simulink model "hvac_1zone_v3"  (R2021a)
settings: Solver=ode45  StartTime=0.0  StopTime=3600*24*3  FixedStep=2  RelTol=1e-3  EnableMultiTasking=on
undefined symbols (not defined in the file or in its folder): den, num, params1, rl
libraries: rllib x1
settings Model: Creator=User  LastModifiedBy=Richi
settings SolverCC: AlgebraicLoopSolver=TrustRegion
settings DataIOCC: LimitDataPoints=on  SaveFormat=Array  SignalLoggingSaveFormat=ModelDataLogs  ReturnWorkspaceOutputs=off
settings OptimizationCC: LifeSpan=inf
settings DebuggingCC: SolverPrmCheckMsg=warning  MultiTaskDSMMsg=warning  MultiTaskCondExecSysMsg=none  MultiTaskRateTransMsg=warning  AllowSymbolicDim=off  SFUnexpectedBacktrackingDiag=warning  SFNoUnconditionalDefaultTransitionDiag=warning  SFExecutionAtInitializationDiag=none  SFMachineParentedDataDiag=warning  ArithmeticOperatorsInVariantConditions=warning
settings HardwareCC: ProdBitPerPointer=32  ProdBitPerSizeT=32  ProdBitPerPtrDiffT=32  ProdLargestAtomicFloat=None  ProdIntDivRoundTo=Undefined  ProdEndianess=Unspecified  ProdWordSize=32  ProdHWDeviceType=32-bit Generic
settings ModelReferenceCC: PropagateSignalLabelsOutOfModel=off
settings SFSimCC: SimUseLocalCustomCode=off  CustomCodeUndefinedFunction=UseInterfaceOnly
settings RTWCC: RTWUseLocalCustomCode=off
settings CodeAppCC: StateflowObjectComments=on
settings GRTTargetCC: TargetLangStandard=C89/C90 (ANSI)
settings ConfigComp: CovMetricSettings=dw  CovSaveCumulativeToWorkspaceVar=on  CovSaveSingleToWorkspaceVar=on  CovExternalEMLEnable=off

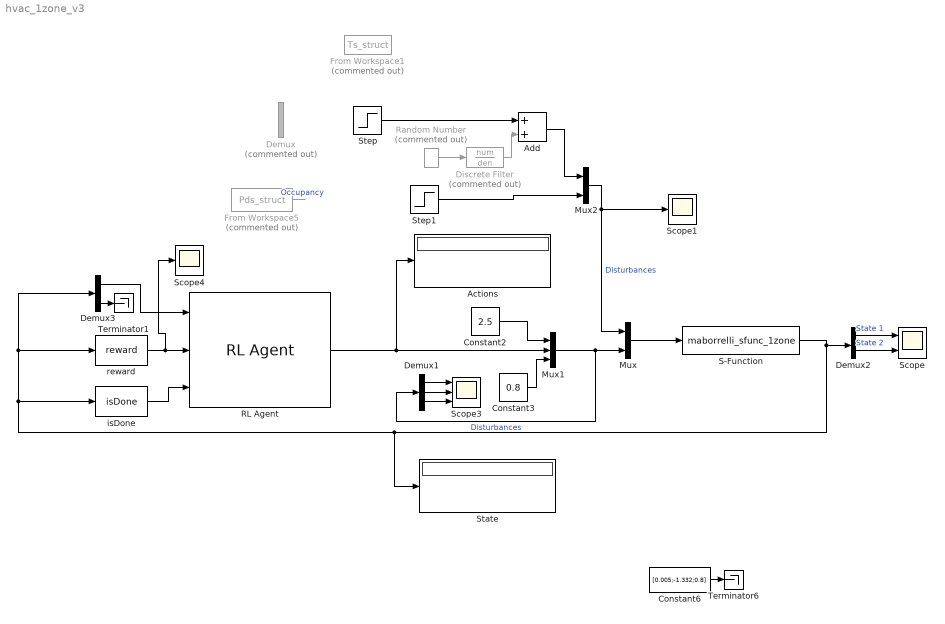
== system hvac_1zone_v3 ==
  Actions : Display
  Add : Sum
  Constant2 : Constant  Value=2.5
  Constant3 : Constant  Value=0.8
  Constant6 : Constant  Value=[0.005;-1.332;0.8]
  Demux : Demux  Commented=on
  Demux1 : Demux  Outputs=3
  Demux2 : Demux  Outputs=2
  Demux3 : Demux  Outputs=2
  Discrete Filter : DiscreteFilter  Commented=on  Numerator=num  Denominator=den  SampleTime=5400
  From Workspace1 : FromWorkspace  Commented=on  VariableName=Ts_struct  OutDataTypeStr=double  SampleTime=-1
  From Workspace5 : FromWorkspace  Commented=on  VariableName=Pds_struct  OutDataTypeStr=double  SampleTime=-1
  Mux : Mux  Inputs=2
  Mux1 : Mux  Inputs=3
  Mux2 : Mux  Inputs=2
  RL Agent : rllib/RL Agent  Agent=rl.util.PolicyInstance.get('hvac_maborrelli_singapur_nzones_with_MPC_v3_manualdist_3/RL Agent')  ExternalActionAsInput=off  ProvideCumRwd=off  TreatAsDirectFeedthrough=on
  Random Number : RandomNumber  Commented=on  Variance=0.5  SampleTime=1800
  S-Function : S-Function  FunctionName=maborrelli_sfunc_1zone  Parameters=[34;34],params1  SFunctionDeploymentMode=off  EnableBusSupport=off
  Scope : Scope  NumInputPorts=2
  Scope1 : Scope
  Scope3 : Scope  NumInputPorts=3
  Scope4 : Scope
  State : Display
  Step : Step  Before=40  After=40  SampleTime=0
  Step1 : Step  Before=200  After=200  SampleTime=0
  Terminator1 : Terminator
  Terminator6 : Terminator
  isDone : M-S-Function  FunctionName=isDone
  reward : M-S-Function  FunctionName=reward
  wires:
  Mux2/1 -> Scope1/1, Mux/1  "Disturbances"
  From Workspace5/1 -> ?  "Occupancy"
  Mux/1 -> S-Function/1
  Constant6/1 -> Terminator6/1
  Discrete Filter/1 -> Add/2
  Add/1 -> Mux2/1
  Random Number/1 -> Discrete Filter/1
  Step/1 -> Add/1
  RL Agent/1 -> Actions/1, Mux1/2
  isDone/1 -> RL Agent/3
  reward/1 -> Scope4/1, RL Agent/2
  S-Function/1 -> Demux2/1, State/1, Demux3/1, reward/1, isDone/1
  Step1/1 -> Mux2/2
  Demux1/2 -> Scope3/2
  Demux1/1 -> Scope3/1
  Demux1/3 -> Scope3/3
  Demux2/1 -> Scope/1  "State 1"
  Demux2/2 -> Scope/2  "State 2"
  Demux3/1 -> RL Agent/1
  Demux3/2 -> Terminator1/1
  Mux1/1 -> Demux1/1, Mux/2  "Disturbances"
  Constant2/1 -> Mux1/1
  Constant3/1 -> Mux1/3
